simulink model "Quad_att_control"  (R2022b)
settings: Solver=ode45  StartTime=0.0  StopTime=10.0  FixedStep=0.001  RelTol=1e-3
values from neighbouring files (symbols this model uses):
  params = containers.Map({'mass','length', 'Inertia', 'k_t', 'k_d', 'g'},{mass, length, I, k_t, k_d, g})    [main.m]    (also in quad_att_control_setup.m)
libraries: slpidlib x3, matrix_library x1, sharedutil x1
settings Model: Creator=dsai9  LastModifiedBy=dsai9

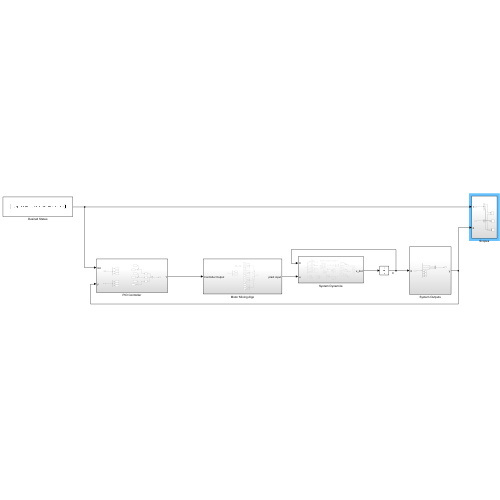
[thumbnail: Simulink's stored preview of the top-level diagram]
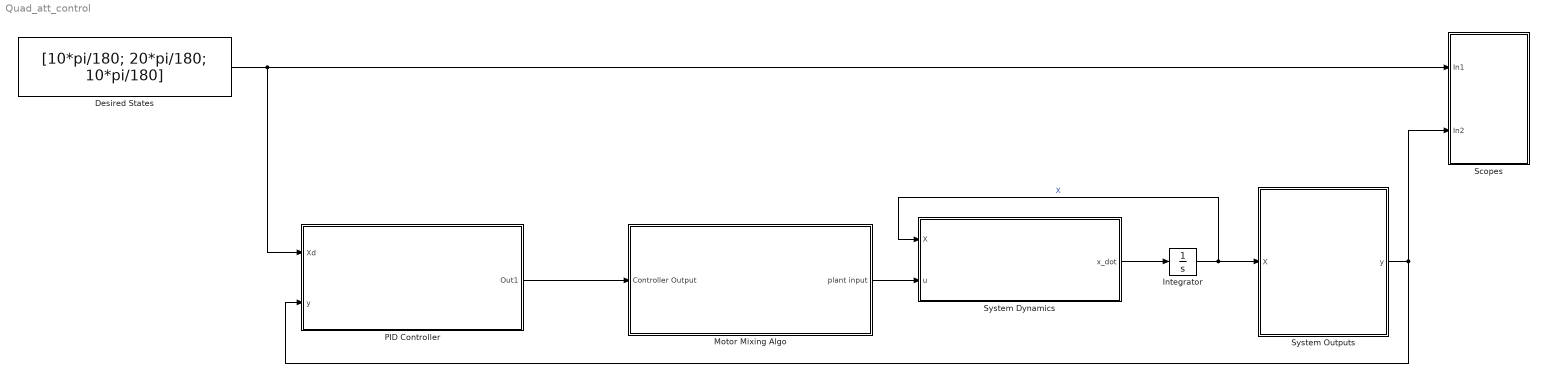
== system Quad_att_control ==
  Desired States : Constant  Value=[10*pi/180; 20*pi/180; 10*pi/180]
  Integrator : Integrator  InitialCondition=[0;0;0;0;0;0]
  Motor Mixing Algo : Subsystem
  PID Controller : Subsystem
  Scopes : Subsystem
  System Dynamics : Subsystem
  System Outputs : Subsystem
  wires:
  System Dynamics/1(x_dot) -> Integrator/1
  Integrator/1 -> System Dynamics/1(X), System Outputs/1(X)  "X"
  Motor Mixing Algo/1(plant input) -> System Dynamics/2(u)
  PID Controller/1(Out1) -> Motor Mixing Algo/1(Controller Output)
  System Outputs/1(y) -> Scopes/2(In2), PID Controller/2(y)
  Desired States/1 -> PID Controller/1(Xd), Scopes/1(In1)

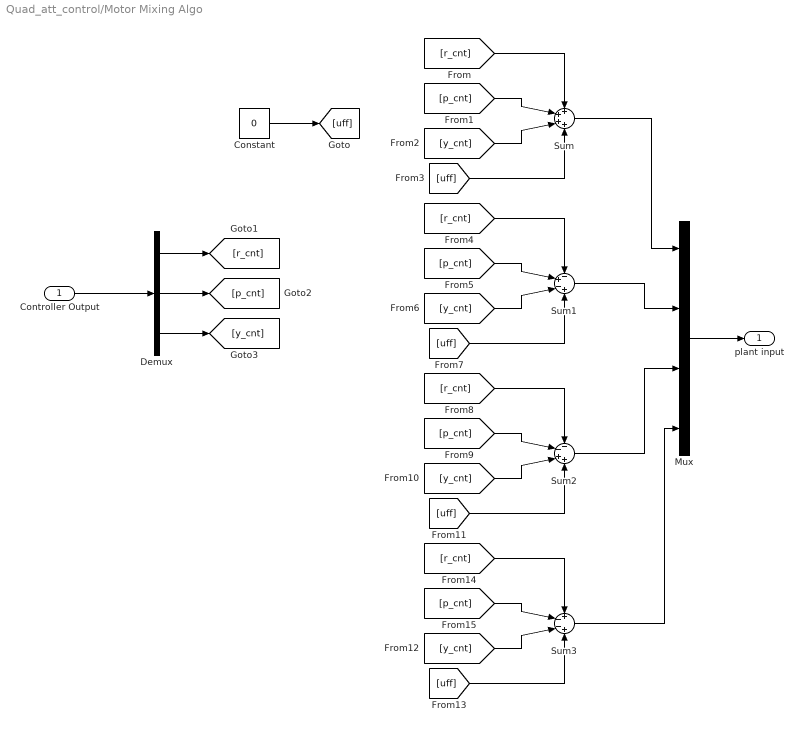
== system Quad_att_control/Motor Mixing Algo ==
  Controller Output : Inport
  Constant : Constant  Value=0
  Demux : Demux  Outputs=3
  Mux : Mux
  Sum : Sum  Inputs=++++
  Sum1 : Sum  Inputs=-+-+
  Sum2 : Sum  Inputs=--++
  Sum3 : Sum  Inputs=+--+
  plant input : Outport
  wires:
  Constant/1 -> [uff]
  Controller Output/1 -> Demux/1
  Demux/1 -> [r_cnt]
  Demux/3 -> [y_cnt]
  Demux/2 -> [p_cnt]
  Mux/1 -> plant input/1
  [r_cnt] -> Sum/1
  [p_cnt] -> Sum/2
  [y_cnt] -> Sum/3
  [uff] -> Sum/4
  Sum/1 -> Mux/1
  Sum1/1 -> Mux/2
  [uff] -> Sum1/4
  [y_cnt] -> Sum1/3
  [p_cnt] -> Sum1/2
  [r_cnt] -> Sum1/1
  [r_cnt] -> Sum2/1
  [p_cnt] -> Sum2/2
  [y_cnt] -> Sum2/3
  [uff] -> Sum2/4
  Sum2/1 -> Mux/3
  Sum3/1 -> Mux/4
  [uff] -> Sum3/4
  [y_cnt] -> Sum3/3
  [p_cnt] -> Sum3/2
  [r_cnt] -> Sum3/1

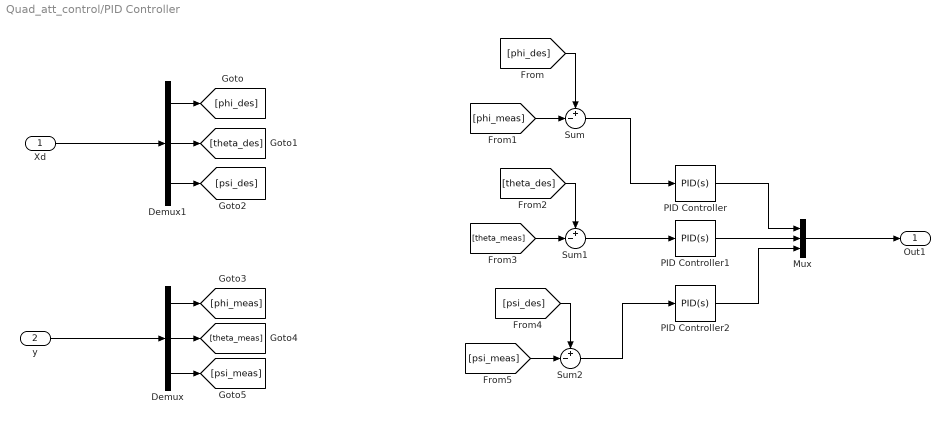
== system Quad_att_control/PID Controller ==
  Xd : Inport
  y : Inport  Port=2
  Demux : Demux  Outputs=3
  Demux1 : Demux  Outputs=3
  Mux : Mux  Inputs=3
  PID Controller : slpidlib/PID Controller  Controller=PID  Form=Parallel  TimeDomain=Continuous-time  UseExternalTs=off  SampleTime=-1  IntegratorMethod=Forward Euler  FilterMethod=Forward Euler  ControllerParametersSource=internal  P=500  I=0  UseKiTs=off  D=300  N=1  UseFilter=on  TunerSelectOption=Transfer Function Based (PID Tuner App)  InitialConditionSource=internal  InitialConditionForIntegrator=0  InitialConditionForFilter=0  DifferentiatorICPrevScaledInput=0  ExternalReset=none  TrackingMode=off  Kt=1  LimitOutput=off  SatLimitsSource=internal  UpperSaturationLimit=inf  LowerSaturationLimit=-inf  LinearizeAsGain=on  AntiWindupMode=none  Kb=1  LimitIntegrator=off  UpperIntegratorSaturationLimit=inf  LowerIntegratorSaturationLimit=-inf  POutMin=[]  POutMax=[]  IOutMin=[]  IOutMax=[]  DOutMin=[]  DOutMax=[]  NOutMin=[]  NOutMax=[]  SumOutMin=[]  SumOutMax=[]  SaturationOutMin=[]  SaturationOutMax=[]  PParamMin=[]  PParamMax=[]  IParamMin=[]  IParamMax=[]  DParamMin=[]  DParamMax=[]  NParamMin=[]  NParamMax=[]  KbParamMin=[]  KbParamMax=[]  KtParamMin=[]  KtParamMax=[]  KbOutMin=[]  KbOutMax=[]  KtOutMin=[]  KtOutMax=[]  IntegratorOutMin=[]  IntegratorOutMax=[]  FilterOutMin=[]  FilterOutMax=[]  SumI1OutMin=[]  SumI1OutMax=[]  SumI2OutMin=[]  SumI2OutMax=[]  SumI3OutMin=[]  SumI3OutMax=[]  SumI4OutMin=[]  SumI4OutMax=[]  SumDOutMin=[]  SumDOutMax=[]  DifferentiatorOutMin=[]  DifferentiatorOutMax=[]  FilterDiffOutCoefMin=[]  FilterDiffOutCoefMax=[]  ReciprocalOutMin=[]  ReciprocalOutMax=[]  SumDenOutMin=[]  SumDenOutMax=[]  SumNumOutMin=[]  SumNumOutMax=[]  DivideOutMin=[]  DivideOutMax=[]  UdiffTsProdOutMin=[]  UdiffTsProdOutMax=[]  NTsProdOutMin=[]  NTsProdOutMax=[]  UintegralTsProdOutMin=[]  UintegralTsProdOutMax=[]  UngainTsProdOutMin=[]  UngainTsProdOutMax=[]  ClampingZeroOutDataTypeStr=Inherit: Inherit via back propagation  ClampingZeroOutMin=[]  ClampingZeroOutMax=[]  FilterDenConstantOutDataTypeStr=Inherit: Inherit via back propagation  FilterDenConstantOutMin=[]  FilterDenConstantOutMax=[]  PCopyOutDataTypeStr=Inherit: Inherit via back propagation  PCopyOutMin=[]  PCopyOutMax=[]  NCopyOutDataTypeStr=Inherit: Inherit via back propagation  NCopyOutMin=[]  NCopyOutMax=[]  IntegratorContinuousStateAttributes=''  IntegratorStateMustResolveToSignalObject=off  IntegratorRTWStateStorageClass=Auto  FilterContinuousStateAttributes=''  FilterStateMustResolveToSignalObject=off  FilterRTWStateStorageClass=Auto  ParallelPVariant=InternalParameters  IdealPVariant=Disabled  IVariant=InternalParameters  DVariant=InternalParameters  IntegratorVariant=Continuous  SatVariant=Disabled  AWVariant=Passthrough  PCopyVariant=Disabled  TRVariant=Disabled  FdbkBlocksVariant=Forward  IdealPFdbkVariant=Disabled  SatFdbkVariant=Disabled  DerivativeFilterVariant=ContFilter  NVariant=InternalParameters  NCopyVariant=Disabled  FilterICVariant=InternalICsFilter  IntegratorICVariant=InternalICs  ExternalResetVariant=Disabled  TRSumVariant=Passthrough  SumFdbkVariant=Disabled  SumVariant=Sum_PID  TsampFilterVariant=InternalTs  TsampNgainVariant=Passthrough  TsampIntegralVariant=Passthrough  ExternalSaturationOutDataTypeStr=Inherit: Same as second input
  PID Controller1 : slpidlib/PID Controller  Controller=PID  Form=Parallel  TimeDomain=Continuous-time  UseExternalTs=off  SampleTime=-1  IntegratorMethod=Forward Euler  FilterMethod=Forward Euler  ControllerParametersSource=internal  P=500  I=0  UseKiTs=off  D=300  N=1  UseFilter=on  TunerSelectOption=Transfer Function Based (PID Tuner App)  InitialConditionSource=internal  InitialConditionForIntegrator=0  InitialConditionForFilter=0  DifferentiatorICPrevScaledInput=0  ExternalReset=none  TrackingMode=off  Kt=1  LimitOutput=off  SatLimitsSource=internal  UpperSaturationLimit=inf  LowerSaturationLimit=-inf  LinearizeAsGain=on  AntiWindupMode=none  Kb=1  LimitIntegrator=off  UpperIntegratorSaturationLimit=inf  LowerIntegratorSaturationLimit=-inf  POutMin=[]  POutMax=[]  IOutMin=[]  IOutMax=[]  DOutMin=[]  DOutMax=[]  NOutMin=[]  NOutMax=[]  SumOutMin=[]  SumOutMax=[]  SaturationOutMin=[]  SaturationOutMax=[]  PParamMin=[]  PParamMax=[]  IParamMin=[]  IParamMax=[]  DParamMin=[]  DParamMax=[]  NParamMin=[]  NParamMax=[]  KbParamMin=[]  KbParamMax=[]  KtParamMin=[]  KtParamMax=[]  KbOutMin=[]  KbOutMax=[]  KtOutMin=[]  KtOutMax=[]  IntegratorOutMin=[]  IntegratorOutMax=[]  FilterOutMin=[]  FilterOutMax=[]  SumI1OutMin=[]  SumI1OutMax=[]  SumI2OutMin=[]  SumI2OutMax=[]  SumI3OutMin=[]  SumI3OutMax=[]  SumI4OutMin=[]  SumI4OutMax=[]  SumDOutMin=[]  SumDOutMax=[]  DifferentiatorOutMin=[]  DifferentiatorOutMax=[]  FilterDiffOutCoefMin=[]  FilterDiffOutCoefMax=[]  ReciprocalOutMin=[]  ReciprocalOutMax=[]  SumDenOutMin=[]  SumDenOutMax=[]  SumNumOutMin=[]  SumNumOutMax=[]  DivideOutMin=[]  DivideOutMax=[]  UdiffTsProdOutMin=[]  UdiffTsProdOutMax=[]  NTsProdOutMin=[]  NTsProdOutMax=[]  UintegralTsProdOutMin=[]  UintegralTsProdOutMax=[]  UngainTsProdOutMin=[]  UngainTsProdOutMax=[]  ClampingZeroOutDataTypeStr=Inherit: Inherit via back propagation  ClampingZeroOutMin=[]  ClampingZeroOutMax=[]  FilterDenConstantOutDataTypeStr=Inherit: Inherit via back propagation  FilterDenConstantOutMin=[]  FilterDenConstantOutMax=[]  PCopyOutDataTypeStr=Inherit: Inherit via back propagation  PCopyOutMin=[]  PCopyOutMax=[]  NCopyOutDataTypeStr=Inherit: Inherit via back propagation  NCopyOutMin=[]  NCopyOutMax=[]  IntegratorContinuousStateAttributes=''  IntegratorStateMustResolveToSignalObject=off  IntegratorRTWStateStorageClass=Auto  FilterContinuousStateAttributes=''  FilterStateMustResolveToSignalObject=off  FilterRTWStateStorageClass=Auto  ParallelPVariant=InternalParameters  IdealPVariant=Disabled  IVariant=InternalParameters  DVariant=InternalParameters  IntegratorVariant=Continuous  SatVariant=Disabled  AWVariant=Passthrough  PCopyVariant=Disabled  TRVariant=Disabled  FdbkBlocksVariant=Forward  IdealPFdbkVariant=Disabled  SatFdbkVariant=Disabled  DerivativeFilterVariant=ContFilter  NVariant=InternalParameters  NCopyVariant=Disabled  FilterICVariant=InternalICsFilter  IntegratorICVariant=InternalICs  ExternalResetVariant=Disabled  TRSumVariant=Passthrough  SumFdbkVariant=Disabled  SumVariant=Sum_PID  TsampFilterVariant=InternalTs  TsampNgainVariant=Passthrough  TsampIntegralVariant=Passthrough  ExternalSaturationOutDataTypeStr=Inherit: Same as second input
  PID Controller2 : slpidlib/PID Controller  Controller=PID  Form=Parallel  TimeDomain=Continuous-time  UseExternalTs=off  SampleTime=-1  IntegratorMethod=Forward Euler  FilterMethod=Forward Euler  ControllerParametersSource=internal  P=3000  I=0  UseKiTs=off  D=3000  N=1  UseFilter=on  TunerSelectOption=Transfer Function Based (PID Tuner App)  InitialConditionSource=internal  InitialConditionForIntegrator=0  InitialConditionForFilter=0  DifferentiatorICPrevScaledInput=0  ExternalReset=none  TrackingMode=off  Kt=1  LimitOutput=off  SatLimitsSource=internal  UpperSaturationLimit=inf  LowerSaturationLimit=-inf  LinearizeAsGain=on  AntiWindupMode=none  Kb=1  LimitIntegrator=off  UpperIntegratorSaturationLimit=inf  LowerIntegratorSaturationLimit=-inf  POutMin=[]  POutMax=[]  IOutMin=[]  IOutMax=[]  DOutMin=[]  DOutMax=[]  NOutMin=[]  NOutMax=[]  SumOutMin=[]  SumOutMax=[]  SaturationOutMin=[]  SaturationOutMax=[]  PParamMin=[]  PParamMax=[]  IParamMin=[]  IParamMax=[]  DParamMin=[]  DParamMax=[]  NParamMin=[]  NParamMax=[]  KbParamMin=[]  KbParamMax=[]  KtParamMin=[]  KtParamMax=[]  KbOutMin=[]  KbOutMax=[]  KtOutMin=[]  KtOutMax=[]  IntegratorOutMin=[]  IntegratorOutMax=[]  FilterOutMin=[]  FilterOutMax=[]  SumI1OutMin=[]  SumI1OutMax=[]  SumI2OutMin=[]  SumI2OutMax=[]  SumI3OutMin=[]  SumI3OutMax=[]  SumI4OutMin=[]  SumI4OutMax=[]  SumDOutMin=[]  SumDOutMax=[]  DifferentiatorOutMin=[]  DifferentiatorOutMax=[]  FilterDiffOutCoefMin=[]  FilterDiffOutCoefMax=[]  ReciprocalOutMin=[]  ReciprocalOutMax=[]  SumDenOutMin=[]  SumDenOutMax=[]  SumNumOutMin=[]  SumNumOutMax=[]  DivideOutMin=[]  DivideOutMax=[]  UdiffTsProdOutMin=[]  UdiffTsProdOutMax=[]  NTsProdOutMin=[]  NTsProdOutMax=[]  UintegralTsProdOutMin=[]  UintegralTsProdOutMax=[]  UngainTsProdOutMin=[]  UngainTsProdOutMax=[]  ClampingZeroOutDataTypeStr=Inherit: Inherit via back propagation  ClampingZeroOutMin=[]  ClampingZeroOutMax=[]  FilterDenConstantOutDataTypeStr=Inherit: Inherit via back propagation  FilterDenConstantOutMin=[]  FilterDenConstantOutMax=[]  PCopyOutDataTypeStr=Inherit: Inherit via back propagation  PCopyOutMin=[]  PCopyOutMax=[]  NCopyOutDataTypeStr=Inherit: Inherit via back propagation  NCopyOutMin=[]  NCopyOutMax=[]  IntegratorContinuousStateAttributes=''  IntegratorStateMustResolveToSignalObject=off  IntegratorRTWStateStorageClass=Auto  FilterContinuousStateAttributes=''  FilterStateMustResolveToSignalObject=off  FilterRTWStateStorageClass=Auto  ParallelPVariant=InternalParameters  IdealPVariant=Disabled  IVariant=InternalParameters  DVariant=InternalParameters  IntegratorVariant=Continuous  SatVariant=Disabled  AWVariant=Passthrough  PCopyVariant=Disabled  TRVariant=Disabled  FdbkBlocksVariant=Forward  IdealPFdbkVariant=Disabled  SatFdbkVariant=Disabled  DerivativeFilterVariant=ContFilter  NVariant=InternalParameters  NCopyVariant=Disabled  FilterICVariant=InternalICsFilter  IntegratorICVariant=InternalICs  ExternalResetVariant=Disabled  TRSumVariant=Passthrough  SumFdbkVariant=Disabled  SumVariant=Sum_PID  TsampFilterVariant=InternalTs  TsampNgainVariant=Passthrough  TsampIntegralVariant=Passthrough  ExternalSaturationOutDataTypeStr=Inherit: Same as second input
  Sum : Sum  Inputs=+-|
  Sum1 : Sum  Inputs=+-|
  Sum2 : Sum  Inputs=+-|
  Out1 : Outport
  wires:
  PID Controller2/1 -> Mux/3
  PID Controller/1 -> Mux/1
  PID Controller1/1 -> Mux/2
  Mux/1 -> Out1/1
  y/1 -> Demux/1
  Xd/1 -> Demux1/1
  Sum/1 -> PID Controller/1
  Demux1/1 -> [phi_des]
  Demux1/2 -> [theta_des]
  Demux1/3 -> [psi_des]
  Demux/1 -> [phi_meas]
  Demux/2 -> [theta_meas]
  Demux/3 -> [psi_meas]
  [phi_des] -> Sum/1
  [phi_meas] -> Sum/2
  [theta_meas] -> Sum1/2
  [theta_des] -> Sum1/1
  Sum1/1 -> PID Controller1/1
  Sum2/1 -> PID Controller2/1
  [psi_des] -> Sum2/1
  [psi_meas] -> Sum2/2

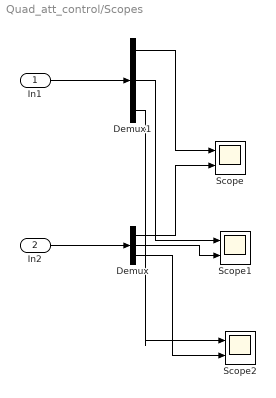
== system Quad_att_control/Scopes ==
  In1 : Inport
  In2 : Inport  Port=2
  Demux : Demux  Outputs=3
  Demux1 : Demux  Outputs=3
  Scope : Scope  NumInputPorts=2
  Scope1 : Scope  NumInputPorts=2
  Scope2 : Scope  NumInputPorts=2
  wires:
  In1/1 -> Demux1/1
  Demux1/1 -> Scope/1
  Demux/3 -> Scope2/2
  Demux/1 -> Scope/2
  In2/1 -> Demux/1
  Demux/2 -> Scope1/2
  Demux1/3 -> Scope2/1
  Demux1/2 -> Scope1/1

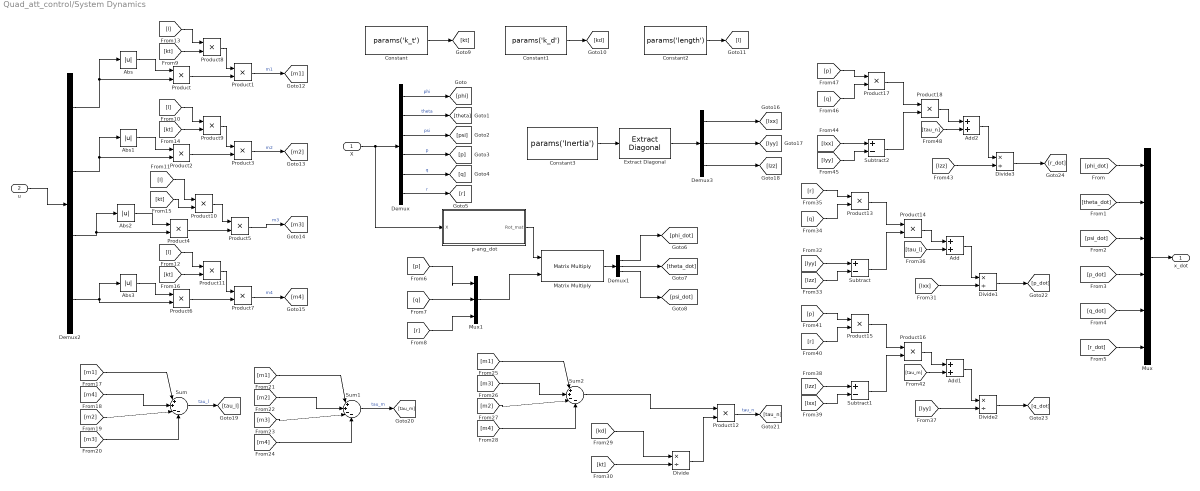
== system Quad_att_control/System Dynamics ==
  X : Inport
  u : Inport  Port=2
  Abs{,1..3} (4 alike) : Abs  SaturateOnIntegerOverflow=off
  Add : Sum
  Add1 : Sum
  Add2 : Sum
  Constant : Constant  Value=params('k_t')
  Constant1 : Constant  Value=params('k_d')
  Constant2 : Constant  Value=params('length')
  Constant3 : Constant  Value=params('Inertia')
  Demux : Demux  Outputs=6
  Demux1 : Demux  Outputs=3
  Demux2 : Demux
  Demux3 : Demux  Outputs=3
  Divide{,1..3} (4 alike) : Product  Inputs=*/
  Extract Diagonal : matrix_library/Extract Diagonal
      settings: LibrarySourceBlock=|
      | simulink/Matrix
      | Operations/Extract Diagonal
  Matrix Multiply : Product  Multiplication=Matrix(*)
  Mux : Mux  Inputs=6
  Mux1 : Mux  Inputs=3
  Product{,1..18} (19 alike) : Product
  Subtract : Sum  Inputs=+-
  Subtract1 : Sum  Inputs=+-
  Subtract2 : Sum  Inputs=+-
  Sum : Sum  Inputs=|++--
  Sum1 : Sum  Inputs=|++--
  Sum2 : Sum  Inputs=|++--
  p-ang_dot : Subsystem
  x_dot : Outport
  wires:
  Demux/4 -> [p]  "p"
  Sum1/1 -> [tau_m]  "tau_m"
  [p] -> Product17/1
  [Ixx] -> Divide1/2
  Demux2/2 -> Abs1/1, Product2/2
  Demux1/1 -> [phi_dot]
  Demux3/2 -> [Iyy]
  X/1 -> p-ang_dot/1(X), Demux/1
  [tau_l] -> Add/2
  Demux2/1 -> Product/2, Abs/1
  [tau_n] -> Add2/2
  [kt] -> Product8/2
  Product12/1 -> [tau_n]  "tau_n"
  Divide3/1 -> [r_dot]
  Abs2/1 -> Product4/1
  [q] -> Product17/2
  Demux/1 -> [phi]  "phi"
  Constant1/1 -> [kd]
  Product11/1 -> Product7/1
  Product10/1 -> Product5/1
  [p_dot] -> Mux/4
  Product15/1 -> Product16/1
  Add2/1 -> Divide3/1
  [q_dot] -> Mux/5
  Sum/1 -> [tau_l]  "tau_l"
  [l] -> Product10/1
  Product17/1 -> Product18/1
  [m4] -> Sum/2
  Product8/1 -> Product1/1
  [p] -> Mux1/1
  [Izz] -> Divide3/2
  [m2] -> Sum/3
  [Ixx] -> Subtract2/1
  Demux/3 -> [psi]  "psi"
  Product18/1 -> Add2/1
  Subtract2/1 -> Product18/2
  Product7/1 -> [m4]  "m4"
  [phi_dot] -> Mux/1
  [l] -> Product8/1
  [Iyy] -> Subtract2/2
  Demux/5 -> [q]  "q"
  [kt] -> Product11/2
  Product2/1 -> Product3/2
  Constant/1 -> [kt]
  [r] -> Mux1/3
  [m3] -> Sum/4
  Demux1/2 -> [theta_dot]
  [kt] -> Product10/2
  [m1] -> Sum/1
  Product/1 -> Product1/2
  p-ang_dot/1(Rot_mat) -> Matrix Multiply/1
  Divide1/1 -> [p_dot]
  Divide/1 -> Product12/2
  Product3/1 -> [m2]  "m2"
  Product16/1 -> Add1/1
  Mux1/1 -> Matrix Multiply/2
  Demux/2 -> [theta]  "theta"
  [psi_dot] -> Mux/3
  [r_dot] -> Mux/6
  Demux1/3 -> [psi_dot]
  [theta_dot] -> Mux/2
  Abs1/1 -> Product2/1
  Subtract/1 -> Product14/2
  Demux/6 -> [r]  "r"
  Demux2/3 -> Product4/2, Abs2/1
  Product4/1 -> Product5/2
  [q] -> Mux1/2
  Constant2/1 -> [l]
  Matrix Multiply/1 -> Demux1/1
  Product14/1 -> Add/1
  Add/1 -> Divide1/1
  Divide2/1 -> [q_dot]
  Add1/1 -> Divide2/1
  [l] -> Product11/1
  [tau_m] -> Add1/2
  Subtract1/1 -> Product16/2
  [r] -> Product15/2
  [Ixx] -> Subtract1/2
  [Iyy] -> Divide2/2
  [Izz] -> Subtract1/1
  [p] -> Product15/1
  Extract Diagonal/1 -> Demux3/1
  [r] -> Product13/1
  Abs/1 -> Product/1
  Product6/1 -> Product7/2
  Demux2/4 -> Abs3/1, Product6/2
  Abs3/1 -> Product6/1
  Product1/1 -> [m1]  "m1"
  Demux3/3 -> [Izz]
  Constant3/1 -> Extract Diagonal/1
  [kd] -> Divide/1
  [kt] -> Product9/2
  Product9/1 -> Product3/1
  [l] -> Product9/1
  [m3] -> Sum1/3
  [m2] -> Sum1/2
  [m4] -> Sum1/4
  [m1] -> Sum1/1
  Product5/1 -> [m3]  "m3"
  u/1 -> Demux2/1
  [m1] -> Sum2/1
  [m3] -> Sum2/2
  [m2] -> Sum2/3
  [m4] -> Sum2/4
  Sum2/1 -> Product12/1
  Product13/1 -> Product14/1
  [q] -> Product13/2
  [kt] -> Divide/2
  [Iyy] -> Subtract/1
  [Izz] -> Subtract/2
  Demux3/1 -> [Ixx]
  Mux/1 -> x_dot/1

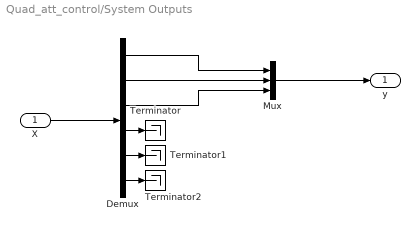
== system Quad_att_control/System Outputs ==
  X : Inport
  Demux : Demux  Outputs=6
  Mux : Mux  Inputs=3
  Terminator : Terminator
  Terminator1 : Terminator
  Terminator2 : Terminator
  y : Outport
  wires:
  Demux/6 -> Terminator2/1
  Demux/4 -> Terminator/1
  Demux/5 -> Terminator1/1
  X/1 -> Demux/1
  Demux/1 -> Mux/1
  Demux/2 -> Mux/2
  Demux/3 -> Mux/3
  Mux/1 -> y/1

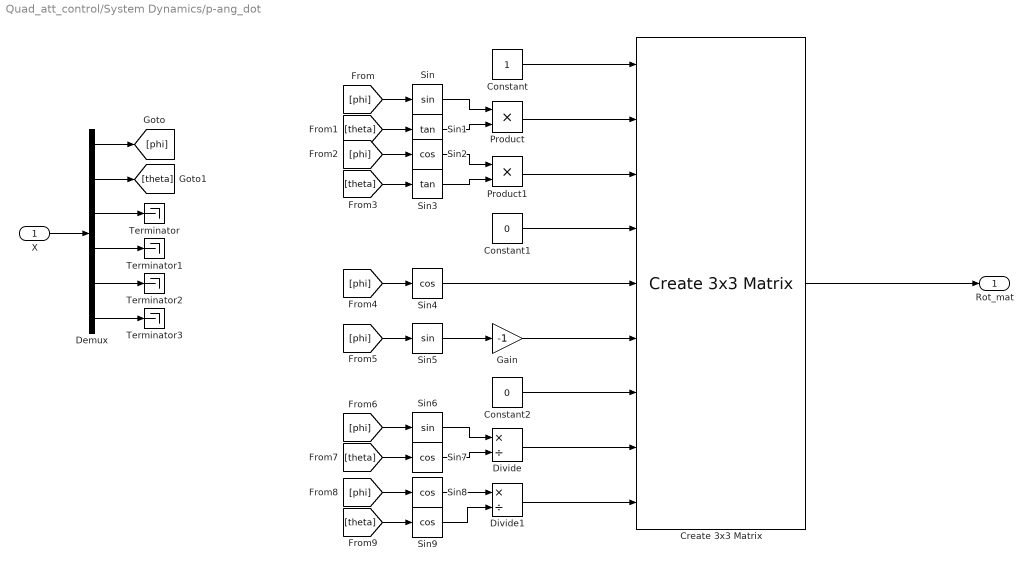
== system Quad_att_control/System Dynamics/p-ang_dot ==
  X : Inport
  Constant : Constant
  Constant1 : Constant  Value=0
  Constant2 : Constant  Value=0
  Create 3x3 Matrix : sharedutil/Create 3x3 Matrix  aMode=aMode
      settings: LibrarySourceBlock=aerolibutil/Create 3x3 Matrix
  Demux : Demux  Outputs=6
  Divide : Product  Inputs=*/  RndMeth=Zero  SaturateOnIntegerOverflow=on
  Divide1 : Product  Inputs=*/  RndMeth=Zero  SaturateOnIntegerOverflow=on
  Gain : Gain  Gain=-1
  Product : Product
  Product1 : Product
  Sin : Trigonometry
  Sin1 : Trigonometry  Operator=tan
  Sin{2,4,7..9} (5 alike) : Trigonometry  Operator=cos
  Sin3 : Trigonometry  Operator=tan
  Sin5 : Trigonometry
  Sin6 : Trigonometry
  Terminator{,1..3} (4 alike) : Terminator
  Rot_mat : Outport
  wires:
  Sin6/1 -> Divide/1
  [phi] -> Sin6/1
  Sin1/1 -> Product/2
  [theta] -> Sin7/1
  Constant2/1 -> Create 3x3 Matrix/7
  Constant/1 -> Create 3x3 Matrix/1
  [theta] -> Sin9/1
  Constant1/1 -> Create 3x3 Matrix/4
  Sin5/1 -> Gain/1
  Sin/1 -> Product/1
  Sin7/1 -> Divide/2
  [phi] -> Sin5/1
  [theta] -> Sin1/1
  Sin8/1 -> Divide1/1
  Gain/1 -> Create 3x3 Matrix/6
  Product/1 -> Create 3x3 Matrix/2
  [phi] -> Sin2/1
  Sin3/1 -> Product1/2
  Sin2/1 -> Product1/1
  Product1/1 -> Create 3x3 Matrix/3
  Divide1/1 -> Create 3x3 Matrix/9
  [theta] -> Sin3/1
  [phi] -> Sin4/1
  [phi] -> Sin/1
  Sin4/1 -> Create 3x3 Matrix/5
  Divide/1 -> Create 3x3 Matrix/8
  [phi] -> Sin8/1
  Sin9/1 -> Divide1/2
  Create 3x3 Matrix/1 -> Rot_mat/1
  X/1 -> Demux/1
  Demux/1 -> [phi]
  Demux/2 -> [theta]
  Demux/3 -> Terminator/1
  Demux/4 -> Terminator1/1
  Demux/5 -> Terminator2/1
  Demux/6 -> Terminator3/1
